simulink model "trav_gyro_PLANT"  (R2022a)
settings: Solver=VariableStepAuto  StartTime=0.0  StopTime=100  RelTol=1e-3
undefined symbols (not defined in the file or in its folder): fix_constg, JLrtg, JMrtg, Kktg, Kvtg
libraries: simulink x4
settings Model: Creator=ohadformanair  LastModifiedBy=ohadformanair
settings SolverCC: MaxConsecutiveMinStep=5  ZeroCrossAlgorithm=Adaptive  MaxZcPerStep=1
settings DebuggingCC: IgnoredZcDiagnostic=none

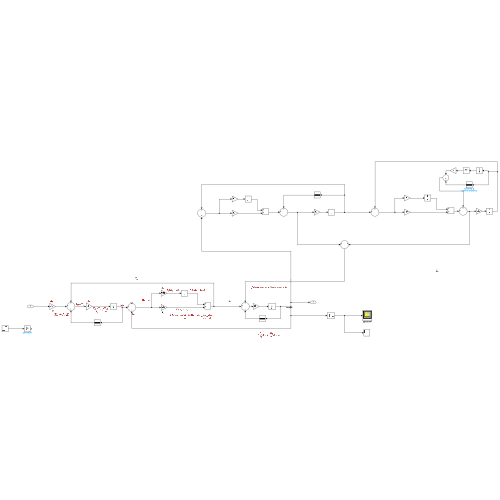
[thumbnail: Simulink's stored preview of the top-level diagram]
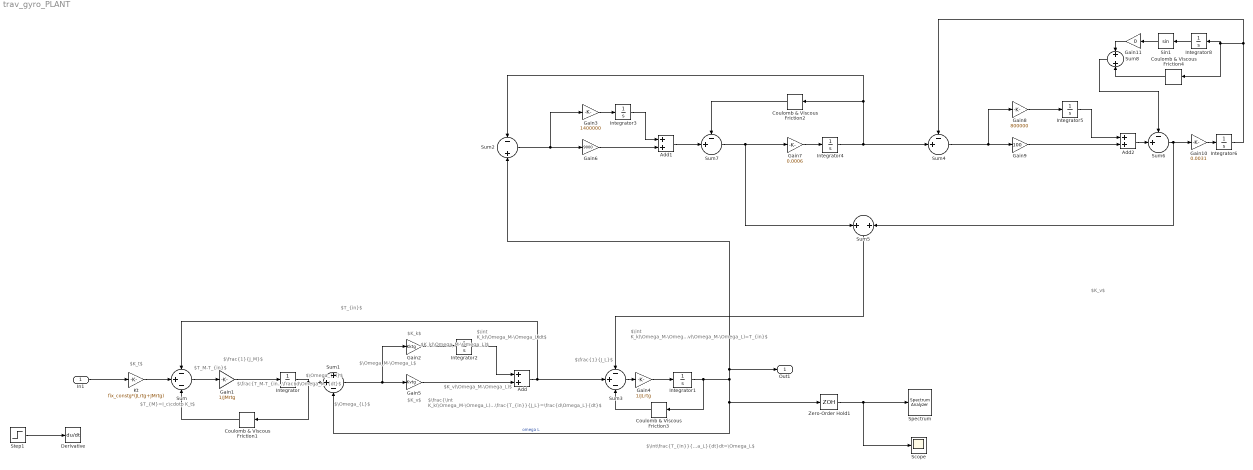
== system trav_gyro_PLANT ==
  note: $\Omega_M-\Omega_L$
  note: $\Omega_{M}$
  note: $T_{in}$
  note: $\Omega_{L}$
  note: $K_v(\Omega_M-\Omega_L)$
  note: $K_v$
  note: $K_k$
  note: $\frac{1}{J_M}$
  note: $\frac{1}{J_L}$
  note: $\int K_k(\Omega_M-\Omega_L)dt$
  note: $K_k(\Omega_M-\Omega_L)$
  note: $\int K_k(\Omega_M-\Omega_L)dt+K_v(\Omega_M-\Omega_L)=T_{in}$
  note: $\frac{\int K_k(\Omega_M-\Omega_L)dt+K_v(\Omega_M-\Omega_L)}{J_L}=\frac{T_{in}}{J_L}=\frac{d\Omega_L}{dt}$
  note: $\int\frac{T_{in}}{J_L}dt=\int\frac{d\Omega_L}{dt}dt=\Omega_L$
  note: $T_{M}=I_c\cdotp K_t$
  note: $K_t$
  note: $T_M-T_{in}$
  note: $\frac{T_M-T_{in}}{J_M}=\frac{d\Omega_M}{dt}$
  note: $K_v$
  In1 : Inport
  Add : Sum
  Add1 : Sum
  Add2 : Sum
  Coulomb & Viscous Friction{1..4} (4 alike) : simulink/Discontinuities/Coulomb & Viscous Friction  offset=0  gain=0
  Derivative : Derivative
  Gain1 : Gain  Gain=1/JMrtg
  Gain10 : Gain  Gain=0.0031
  Gain11 : Gain  Gain=0
  Gain2 : Gain  Gain=Kktg
  Gain3 : Gain  Gain=1400000
  Gain4 : Gain  Gain=1/JLrtg
  Gain5 : Gain  Gain=Kvtg
  Gain6 : Gain  Gain=9000
  Gain7 : Gain  Gain=0.0006
  Gain8 : Gain  Gain=800000
  Gain9 : Gain  Gain=100
  Integrator{,1..6,8} (8 alike) : Integrator
  Kt : Gain  Gain=fix_constg*(JLrtg+JMrtg)
  Scope : Scope
  Sin1 : Trigonometry
  "Spectrum " : SpectrumAnalyzer
  Step1 : Step  SampleTime=0
  Sum : Sum  Inputs=-+-
  Sum1 : Sum  Inputs=++-
  Sum2 : Sum  Inputs=-+
  Sum3 : Sum  Inputs=-+-
  Sum4 : Sum  Inputs=-+|
  Sum5 : Sum
  Sum6 : Sum  Inputs=-+|
  Sum7 : Sum  Inputs=-+|
  Sum8 : Sum
  Zero-Order Hold1 : ZeroOrderHold  SampleTime=0.005
  Out1 : Outport
  wires:
  Kt/1 -> Sum/2
  Gain4/1 -> Integrator1/1
  Sum/1 -> Gain1/1
  Gain1/1 -> Integrator/1
  Integrator/1 -> Coulomb & Viscous Friction1/1, Sum1/2
  Integrator1/1 -> Coulomb & Viscous Friction3/1, Zero-Order Hold1/1, Sum1/3, Out1/1, Sum2/2  "omega L"
  Integrator2/1 -> Add/1
  Sum1/1 -> Gain5/1, Gain2/1
  Gain2/1 -> Integrator2/1
  Gain5/1 -> Add/2
  Add/1 -> Sum3/2, Sum/1
  Gain6/1 -> Add1/2
  Integrator3/1 -> Add1/1
  Sum2/1 -> Gain6/1, Gain3/1
  Gain3/1 -> Integrator3/1
  Gain7/1 -> Integrator4/1
  Sum3/1 -> Gain4/1
  Integrator5/1 -> Add2/1
  Gain9/1 -> Add2/2
  Gain8/1 -> Integrator5/1
  Sum4/1 -> Gain9/1, Gain8/1
  Gain10/1 -> Integrator6/1
  Integrator6/1 -> Coulomb & Viscous Friction4/1, Integrator8/1, Sum4/1
  Sum5/1 -> Sum3/1
  Integrator4/1 -> Sum4/2, Coulomb & Viscous Friction2/1, Sum2/1
  Add2/1 -> Sum6/2
  Sum6/1 -> Sum5/2, Gain10/1
  Add1/1 -> Sum7/2
  Sum7/1 -> Gain7/1, Sum5/1
  Coulomb & Viscous Friction1/1 -> Sum/3
  Coulomb & Viscous Friction2/1 -> Sum7/1
  Coulomb & Viscous Friction3/1 -> Sum3/3
  Coulomb & Viscous Friction4/1 -> Sum8/2
  Sin1/1 -> Gain11/1
  Integrator8/1 -> Sin1/1
  Gain11/1 -> Sum8/1
  Sum8/1 -> Sum6/1
  Step1/1 -> Derivative/1
  Zero-Order Hold1/1 -> Scope/1, "Spectrum "/1
  In1/1 -> Kt/1
